simulink model "truck"  (R2022a)
(part 5 of 17)

  M5_erp33360_kros_i_takviyeler_IGS_4_RIGID/LConn1 -- Transform164/RConn1
  M5_erpAynalama3360_kulak_i_takviye_IGS_2_RIGID/LConn1 -- Transform165/RConn1
  M5_erpAynalamaAynalama33360_Kulak_i_L_takviye_IGS_1_RIGID/LConn1 -- Transform166/RConn1
  M5_erp33360_takviye_1_IGS_2_RIGID/LConn1 -- Transform167/RConn1
  M5_erpAynalama33360_kros_ke_takviye_IGS_1_RIGID/LConn1 -- Transform168/RConn1
  M5_erpAynalama33360_kanca_IGS_9_RIGID/LConn1 -- Transform169/RConn1
  Transform17/RConn1 -- mandud_ase_arka_i_destek_1_IGS_1_RIGID/LConn1
  M5_erp33360_takviye_3_IGS_1_RIGID/LConn1 -- Transform170/RConn1
  M5_erp33360_takviye_2_IGS_2_RIGID/LConn1 -- Transform171/RConn1
  M5_erpAynalama33360_kanca_IGS_8_RIGID/LConn1 -- Transform172/RConn1
  M5_erp33360_takviye_2_IGS_1_RIGID/LConn1 -- Transform173/RConn1
  M5_erp33360_takviye_1_IGS_3_RIGID/LConn1 -- Transform174/RConn1
  M5_erpAynalama33360_takviye_3_IGS_1_RIGID/LConn1 -- Transform175/RConn1
  M5_erp3360_kulak_i_takviye_IGS_1_RIGID/LConn1 -- Transform176/RConn1
  M5_erpAynalama33360_takviye_1_IGS_2_RIGID/LConn1 -- Transform177/RConn1
  M5_erp33360_takviye_1_IGS_1_RIGID/LConn1 -- Transform178/RConn1
  M5_erpAynalama33360_takviye_1_IGS_1_RIGID/LConn1 -- Transform179/RConn1
  Transform18/RConn1 -- mandUD_yan_lamba_kablo_borusu_IGS_4_RIGID/LConn1
  M5_erpAynalama33360_takviye_2_IGS_1_RIGID/LConn1 -- Transform180/RConn1
  M5_erpAynalama33360_takviye_2_IGS_2_RIGID/LConn1 -- Transform181/RConn1
  M5_erp33360_kros_ke_takviye_IGS_1_RIGID/LConn1 -- Transform182/RConn1
  M5_erp33360_kros_ke_takviye_IGS_3_RIGID/LConn1 -- Transform183/RConn1
  M5_erp33360_kros_i_takviyeler_IGS_1_RIGID/LConn1 -- Transform184/RConn1
  M5_erp33360_kros_i_takviyeler_IGS_2_RIGID/LConn1 -- Transform185/RConn1
  M5_erp33360_kros_i_takviyeler_IGS_3_RIGID/LConn1 -- Transform186/RConn1
  M5_erp33360_kros_ke_takviye_IGS_4_RIGID/LConn1 -- Transform187/RConn1
  M5_erp33360_merdiven_kula_IGS_2_RIGID/LConn1 -- Transform188/RConn1
  M5_erp33360_merdiven_kula_IGS_5_RIGID/LConn1 -- Transform189/RConn1
  Transform19/RConn1 -- mandud_ase_arka_i_destek_2_IGS_1_RIGID/LConn1
  M5_erpAynalama33360_kros_i_takviyeler_IGS_3_RIGID/LConn1 -- Transform190/RConn1
  M5_erp33360_basamak_IGS_4_RIGID/LConn1 -- Transform191/RConn1
  M5_erp33360_mapa_IGS_2_RIGID/LConn1 -- Transform192/RConn1
  M5_erpAynalama33360_mapa_IGS_2_RIGID/LConn1 -- Transform193/RConn1
  AynalamaM5_erp33360_ZBEKSTAN_ngs_kuak_krosu_IGS_1_RIGID/LConn1 -- Transform194/RConn1
  M5_erp33360_merdiven_kula_IGS_1_RIGID/LConn1 -- Transform195/RConn1
  M5_erp33360_Emniyet_kolu_kasa_paras2_IGS_2_RIGID/LConn1 -- Transform196/RConn1
  M5_erp33360_basamak_IGS_3_RIGID/LConn1 -- Transform197/RConn1
  M5_erp33360_merdiven_kula_IGS_4_RIGID/LConn1 -- Transform198/RConn1
  M5_erpAynalama33360_kros_i_takviyeler_IGS_4_RIGID/LConn1 -- Transform199/RConn1
  Transform2/RConn1 -- x33360_33360_esnek_V_st_para_IGS_1_RIGID/LConn1
  Transform20/RConn1 -- manasi_flan_k8_4_IGS_1_RIGID/LConn1
  M5_erp33360_basamak_IGS_2_RIGID/LConn1 -- Transform200/RConn1
  M5_erp33360_basamak_IGS_5_RIGID/LConn1 -- Transform201/RConn1
  M5_erp33360_merdiven_kenar_IGS_1_RIGID/LConn1 -- Transform202/RConn1
  M5_erp33360_basamak_IGS_6_RIGID/LConn1 -- Transform203/RConn1
  M5_erp33360_basamak_IGS_1_RIGID/LConn1 -- Transform204/RConn1
  M5_erp33360_Emniyet_kolu_kasa_paras1_IGS_1_RIGID/LConn1 -- Transform205/RConn1
  M5_erpAynalama33360_kros_ke_takviye_IGS_2_RIGID/LConn1 -- Transform206/RConn1
  M5_erpAynalama33360_kros_i_takviyeler_IGS_1_RIGID/LConn1 -- Transform207/RConn1
  M5_erpAynalama33360_kros_i_takviyeler_IGS_2_RIGID/LConn1 -- Transform208/RConn1
  M5_erp33360_merdiven_kenar_IGS_2_RIGID/LConn1 -- Transform209/RConn1
  Transform21/RConn1 -- manasi_flan_k8_4_IGS_3_RIGID/LConn1
  M5_erp33360_basamak_IGS_7_RIGID/LConn1 -- Transform210/RConn1
  M5_erp33360_basamak_IGS_8_RIGID/LConn1 -- Transform211/RConn1
  M5_erp33360_merdiven_kula_IGS_3_RIGID/LConn1 -- Transform212/RConn1
  M5_erp33360_Emniyet_kolu_kasa_paras2_IGS_1_RIGID/LConn1 -- Transform213/RConn1
  M5_erp33360_merdiven_kula_IGS_6_RIGID/LConn1 -- Transform214/RConn1
  M5_erp33360_mapa_IGS_1_RIGID/LConn1 -- Transform215/RConn1
  M5_erpAynalama33360_mapa_IGS_1_RIGID/LConn1 -- Transform216/RConn1
  AynalamaM5_erp33360_ZBEKSTAN_kk_yan_kros_IGS_1_RIGID/LConn1 -- Transform217/RConn1
  Kopya_MA_Part_PISTON_GHS_175_5_5550_CM5_Model_004_merkez_IGS_1_/LConn1 -- Transform218/RConn1
  M5_erp33360_n_arka_amurluk_Yeni_Tip_k3_IGS_1_RIGID/LConn1 -- Transform219/RConn1
  Transform22/RConn1 -- manasi_flan_k8_4_IGS_4_RIGID/LConn1
  M5_erp33360_siperlik_IGS_1_RIGID/LConn1 -- Transform220/RConn1
  M5_erp33360_KMS_298_IGS_1_RIGID/LConn1 -- Transform221/RConn1
  M5_erp33360_Aynalamaamurluk_aya_kebenti_6mm_IGS_3_RIGID/LConn1 -- Transform222/RConn1
  M5_erp33360_amurluk_aya_kebenti_6mm_IGS_1_RIGID/LConn1 -- Transform223/RConn1
  M5_erp33360_KMS_207_IGS_1_RIGID/LConn1 -- Transform224/RConn1
  M5_erp33360_Aynalamaamurluk_aya_kebenti_6mm_IGS_4_RIGID/LConn1 -- Transform225/RConn1
  M5_erp33360_KMS_298_IGS_2_RIGID/LConn1 -- Transform226/RConn1
  M5_erp33360_Aynalamai_kaytr_IGS_1_RIGID/LConn1 -- Transform227/RConn1
  M5_erp33360_KMK_226_IGS_1_RIGID/LConn1 -- Transform228/RConn1
  M5_erp33360_ase_kamaz_6_mm_IGS_1_RIGID/LConn1 -- Transform229/RConn1
  Transform23/RConn1 -- manasi_flan_k8_4_IGS_2_RIGID/LConn1
  M5_erp33360_KMS_202_IGS_2_RIGID/LConn1 -- Transform230/RConn1
  M5_erp33360_KMS_202_IGS_3_RIGID/LConn1 -- Transform231/RConn1
  M5_erp33360_siperlik_yan_sac_IGS_1_RIGID/LConn1 -- Transform232/RConn1
  M5_erp33360_KMS_202_IGS_1_RIGID/LConn1 -- Transform233/RConn1
  M5_erp33360_Aynalamaamurluk_aya_kebenti_6mm_IGS_2_RIGID/LConn1 -- Transform234/RConn1
  M5_erp33360_ase_kamaz_6_mm_IGS_2_RIGID/LConn1 -- Transform235/RConn1
  M5_erp33360_Aynalamasiperlik_yan_sac_IGS_1_RIGID/LConn1 -- Transform236/RConn1
  M5_erp33360_KMS_202_IGS_4_RIGID/LConn1 -- Transform237/RConn1
  M5_erp33360_kros_kebent_IGS_1_RIGID/LConn1 -- Transform238/RConn1
  M5_erp33360_amurluk_aya_kk_kebent_6mm_IGS_1_RIGID/LConn1 -- Transform239/RConn1
  Transform24/RConn1 -- manpistonaltbaskstsac_k10_1_IGS_1_RIGID/LConn1
  M5_erp33360_Aynalamaamurluk_aya_kebenti_6mm_IGS_1_RIGID/LConn1 -- Transform240/RConn1
  M5_erp33360_HD_654_IGS_1_RIGID/LConn1 -- Transform241/RConn1
  M5_erp33360_ase_kamaz_arka_sac_6mm_IGS_1_RIGID/LConn1 -- Transform242/RConn1
  M5_erpAynalama33360_KMS_202_IGS_2_RIGID/LConn1 -- Transform243/RConn1
  M5_erpAynalama33360_KMS_202_IGS_4_RIGID/LConn1 -- Transform244/RConn1
  M5_erpAynalama33360_KMK_236_IGS_1_RIGID/LConn1 -- Transform245/RConn1
  M5_erp33360_siperlik_lamas_IGS_1_RIGID/LConn1 -- Transform246/RConn1
  M5_erpAynalama33360_KMS_207_IGS_1_RIGID/LConn1 -- Transform247/RConn1
  M5_erpAynalama33360_Aynalamaamurluk_aya_kebenti_6mm_IGS_1_RIGID/LConn1 -- Transform248/RConn1
  M5_erpAynalama33360_amurluk_sac_k4_IGS_1_RIGID/LConn1 -- Transform249/RConn1
  Transform25/RConn1 -- mandAynalamaUD_altbask_i_IGS_1_RIGID/LConn1
  M5_erp33360_Aynalamanpanel_dke_takviyesi_IGS_1_RIGID/LConn1 -- Transform250/RConn1
  M5_erpAynalama33360_KMS_202_IGS_3_RIGID/LConn1 -- Transform251/RConn1
  M5_erpAynalama33360_KMS_202_IGS_1_RIGID/LConn1 -- Transform252/RConn1
  M5_erp33360_npanel_dke_takviyesi_IGS_1_RIGID/LConn1 -- Transform253/RConn1
  M5_erpAynalama33360_i_amurluk_aya_k6_IGS_2_RIGID/LConn1 -- Transform254/RConn1
  M5_erpAynalama33360_i_amurluk_aya_paspas_gelenler_IGS_1_RIGID/LConn1 -- Transform255/RConn1
  M5_erpAynalama33360_n_arka_amurluk_Yeni_Tip_k3_IGS_1_RIGID/LConn1 -- Transform256/RConn1
  M5_erp33360_i_sehim_takviyesi_IGS_1_RIGID/LConn1 -- Transform257/RConn1
  M5_erpAynalama33360_i_amurluk_aya_k6_IGS_1_RIGID/LConn1 -- Transform258/RConn1
  M5_erp33360_npanel_ike_takviyesi_IGS_1_RIGID/LConn1 -- Transform259/RConn1
  Transform26/RConn1 -- mandUD_altbask_i_IGS_1_RIGID/LConn1
  M5_erpAynalama33360_n_amurluk_aya_k6_IGS_1_RIGID/LConn1 -- Transform260/RConn1
  M5_erpAynalama33360_npanel_ike_takviyesi_IGS_1_RIGID/LConn1 -- Transform261/RConn1
  M5_erp33360_n_arka_amurluk_Yeni_Tip_k3_IGS_2_RIGID/LConn1 -- Transform262/RConn1
  M5_erp33360_i_sehim_takviyesi_IGS_2_RIGID/LConn1 -- Transform263/RConn1
  M5_erpAynalama33360_arka_amurluk_aya_6mm_IGS_1_RIGID/LConn1 -- Transform264/RConn1
  M5_erpAynalama33360_i_amurluk_aya_paspas_gelenler_IGS_2_RIGID/LConn1 -- Transform265/RConn1
  M5_erpAynalama33360_n_arka_amurluk_Yeni_Tip_k3_IGS_2_RIGID/LConn1 -- Transform266/RConn1
  M5_erpAynalama33360_HD_654_IGS_1_RIGID/LConn1 -- Transform267/RConn1
  M5_erpAynalama33360_KMK_226_IGS_1_RIGID/LConn1 -- Transform268/RConn1
  M5_erpAynalama33360_KMS_298_IGS_1_RIGID/LConn1 -- Transform269/RConn1
  Transform27/RConn1 -- mandUD_ya_tank_aya_destek_IGS_1_RIGID/LConn1
  M5_erpAynalama33360_KMS_298_IGS_2_RIGID/LConn1 -- Transform270/RConn1
  M5_erpAynalama33360_kros_kebent_IGS_1_RIGID/LConn1 -- Transform271/RConn1
  M5_erpAynalama33360_Aynalamaamurluk_aya_kebenti_6mm_IGS_2_RIGID/LConn1 -- Transform272/RConn1
  M5_erpAynalama33360_amurluk_aya_kk_kebent_6mm_IGS_1_RIGID/LConn1 -- Transform273/RConn1
  M5_erpAynalama33360_ase_kamaz_6_mm_IGS_1_RIGID/LConn1 -- Transform274/RConn1
  M5_erpAynalama33360_ase_kamaz_arka_sac_6mm_IGS_1_RIGID/LConn1 -- Transform275/RConn1
  M5_erpAynalama33360_Aynalamaamurluk_aya_kebenti_6mm_IGS_4_RIGID/LConn1 -- Transform276/RConn1
  M5_erpAynalama33360_amurluk_aya_kebenti_6mm_IGS_1_RIGID/LConn1 -- Transform277/RConn1
  M5_erp33360_ikayt_arka_kaama_IGS_1_RIGID/LConn1 -- Transform278/RConn1
  M5_erpAynalama33360_ikayt_arka_kaama_IGS_1_RIGID/LConn1 -- Transform279/RConn1
  Transform28/RConn1 -- mandUD_yan_lamba_kablo_borusu_IGS_1_RIGID/LConn1
  M5_erpAynalama33360_ase_kamaz_6_mm_IGS_2_RIGID/LConn1 -- Transform280/RConn1
  M5_erp33360_kapak_IGS_1_RIGID/LConn1 -- Transform281/RConn1
  M5_erpAynalama33360_Aynalamaamurluk_aya_kebenti_6mm_IGS_3_RIGID/LConn1 -- Transform282/RConn1
  Transform283/RConn1 -- x33360_pulll_IGS_9_RIGID/LConn1
  Transform284/RConn1 -- x33360_33360_esnek_V_st_para_IGS_2_RIGID/LConn1
  Transform285/RConn1 -- x33360_pulll_IGS_12_RIGID/LConn1
  Transform286/RConn1 -- x33360_23658911_IGS_3_RIGID/LConn1
  Transform287/RConn1 -- x33360_23658911_IGS_5_RIGID/LConn1
  Transform288/RConn1 -- x33360_23658911_IGS_7_RIGID/LConn1
  Transform289/RConn1 -- x33360_esnek_baglanti_poliuretan_takoz_IGS_2_RIGID/LConn1
  Transform29/RConn1 -- ayakflan_k8_4_IGS_2_RIGID/LConn1
  Transform290/RConn1 -- x33360_33360_2li_esnke_ara_para_IGS_2_RIGID/LConn1
  Transform291/RConn1 -- x33360_HEX_NUT_ISO_8673_M16_X_1_5_IGS_3_RIGID/LConn1
  Transform292/RConn1 -- x33360_23658911_IGS_6_RIGID/LConn1
  Transform293/RConn1 -- x33360_33360_2li_esnke_ara_para_IGS_1_RIGID/LConn1
  Transform294/RConn1 -- x33360_pulll_IGS_2_RIGID/LConn1
  Transform295/RConn1 -- x33360_pulll_IGS_4_RIGID/LConn1
  Transform296/RConn1 -- x33360_pulll_IGS_8_RIGID/LConn1
  Transform297/RConn1 -- x33360_33360_esnek_ust_ped_IGS_1_RIGID/LConn1
  Transform298/RConn1 -- x33360_pulll_IGS_6_RIGID/LConn1
  Transform299/RConn1 -- x33360_33360_Esnek_V_alt_para_uzun_IGS_1_RIGID/LConn1
  M33360_26280_mil_no8_IGS_1_RIGID/LConn1 -- Transform3/RConn1
  Transform30/RConn1 -- ayakflan_k8_4_IGS_3_RIGID/LConn1
  Transform300/RConn1 -- x33360_pulll_IGS_3_RIGID/LConn1
  Transform301/RConn1 -- x33360_33360_esnek_ust_ped_IGS_2_RIGID/LConn1
  Transform302/RConn1 -- x33360_pulll_IGS_5_RIGID/LConn1
  Transform303/RConn1 -- x33360_pulll_IGS_7_RIGID/LConn1
  Transform304/RConn1 -- x33360_33360_ESNEK_UZUN_ALT_PED_IGS_1_RIGID/LConn1
  Transform305/RConn1 -- x33360_pulll_IGS_10_RIGID/LConn1
  Transform306/RConn1 -- x33360_pulll_IGS_1_RIGID/LConn1
  Transform307/RConn1 -- x33360_pulll_IGS_11_RIGID/LConn1
  Transform308/RConn1 -- x33360_23658911_IGS_1_RIGID/LConn1
  Transform309/RConn1 -- x33360_23658911_IGS_2_RIGID/LConn1
  Transform31/RConn1 -- x132zbmut4900zT13124_ozaas_Part2_IGS_1_RIGID/LConn1
  Transform310/RConn1 -- x33360_23658911_IGS_4_RIGID/LConn1
  Transform311/RConn1 -- x33360_23658911_IGS_8_RIGID/LConn1
  Transform312/RConn1 -- x33360_esnek_baglanti_poliuretan_takoz_IGS_1_RIGID/LConn1
  Transform313/RConn1 -- x33360_HEX_NUT_ISO_8673_M16_X_1_5_IGS_1_RIGID/LConn1
  Transform314/RConn1 -- x33360_HEX_NUT_ISO_8673_M16_X_1_5_IGS_2_RIGID/LConn1
  Aynalama33360_33360_esnek_V_st_para_IGS_2_RIGID/LConn1 -- Transform315/RConn1
  Transform316/RConn1 -- x33360_burlu_balant_burcu_IGS_2_RIGID/LConn1
  Aynalama33360_pulll_IGS_1_RIGID/LConn1 -- Transform317/RConn1
  Transform318/RConn1 -- x33360_HEX_NUT_ISO_8673_M16_X_1_5_IGS_4_RIGID/LConn1
  Aynalama33360_33360_2li_esnke_ara_para_IGS_2_RIGID/LConn1 -- Transform319/RConn1
  Transform32/RConn1 -- x132zbmut4900zT13124_ozaas_Part2_IGS_2_RIGID/LConn1
  Aynalama33360_pulll_IGS_8_RIGID/LConn1 -- Transform320/RConn1
  Aynalama33360_pulll_IGS_5_RIGID/LConn1 -- Transform321/RConn1
  Transform322/RConn1 -- x33360_KMS_305_IGS_1_RIGID/LConn1
  Son_model_3_IGS_3_RIGID/LConn1 -- Transform323/RConn1
  Aynalama33360_esnek_baglanti_poliuretan_takoz_IGS_1_RIGID/LConn1 -- Transform324/RConn1
  Transform325/RConn1 -- x33360_MS_009_IGS_1_RIGID/LConn1
  Aynalama33360_pulll_IGS_2_RIGID/LConn1 -- Transform326/RConn1
  Aynalama33360_esnek_baglanti_poliuretan_takoz_IGS_2_RIGID/LConn1 -- Transform327/RConn1
  Aynalama33360_pulll_IGS_11_RIGID/LConn1 -- Transform328/RConn1
  Transform329/RConn1 -- x33360_burlu_balant_burcu_IGS_1_RIGID/LConn1
  Ayak_Sac3_752_IGS_1_RIGID/LConn1 -- Transform33/RConn1
  Aynalama33360_33360_Esnek_V_alt_para_uzun_IGS_1_RIGID/LConn1 -- Transform330/RConn1
  Aynalama33360_33360_2li_esnke_ara_para_IGS_1_RIGID/LConn1 -- Transform331/RConn1
  Aynalama33360_33360_esnek_ust_ped_IGS_2_RIGID/LConn1 -- Transform332/RConn1
  Transform333/RConn1 -- x33360_arkamilbalant_IGS_1_RIGID/LConn1
  Son_model_3_IGS_1_RIGID/LConn1 -- Transform334/RConn1
  Aynalama33360_33360_ESNEK_UZUN_ALT_PED_IGS_1_RIGID/LConn1 -- Transform335/RConn1
  Transform336/RConn1 -- x33360_MS_008_IGS_1_RIGID/LConn1
  Son_model_3_IGS_2_RIGID/LConn1 -- Transform337/RConn1
  Aynalama33360_33360_esnek_V_st_para_IGS_1_RIGID/LConn1 -- Transform338/RConn1
  Aynalama33360_33360_esnek_ust_ped_IGS_1_RIGID/LConn1 -- Transform339/RConn1
  Transform34/RConn1 -- ayakflan_k8_4_IGS_1_RIGID/LConn1
  Aynalama33360_pulll_IGS_3_RIGID/LConn1 -- Transform340/RConn1
  Aynalama33360_pulll_IGS_4_RIGID/LConn1 -- Transform341/RConn1
  Aynalama33360_pulll_IGS_6_RIGID/LConn1 -- Transform342/RConn1
  Aynalama33360_pulll_IGS_7_RIGID/LConn1 -- Transform343/RConn1
  Aynalama33360_pulll_IGS_9_RIGID/LConn1 -- Transform344/RConn1
  Aynalama33360_pulll_IGS_10_RIGID/LConn1 -- Transform345/RConn1
  Aynalama33360_pulll_IGS_12_RIGID/LConn1 -- Transform346/RConn1
  Aynalama33360_HEX_NUT_ISO_8673_M16_X_1_5_IGS_4_RIGID/LConn1 -- Transform347/RConn1
  Transform348/RConn1 -- st_kapama_L_ayak_sasi_paras_21_IGS_2_RIGID/LConn1
  AynalamaSon_model_3_IGS_1_RIGID/LConn1 -- Transform349/RConn1
  Ayak_Sac4_692_IGS_1_RIGID/LConn1 -- Transform35/RConn1
  Transform350/RConn1 -- ayakl_flans_IGS_1_RIGID/LConn1
  Ayak_U_ase_paras_IGS_1_RIGID/LConn1 -- Transform351/RConn1
  Transform352/RConn1 -- st_kapama_L_ayak_sasi_paras_21_IGS_1_RIGID/LConn1
  Transform353/RConn1 -- YAPI_plastik_cmurluk_bru_ust_bayrak_IGS_2_RIGID/LConn1
  Aynalama33360_MS_008_IGS_1_RIGID/LConn1 -- Transform354/RConn1
  AynalamaYAPI_plastik_cmurluk_bru_ust_bayrak_IGS_4_RIGID/LConn1 -- Transform355/RConn1
  AynalamaYAPI_plastik_camurluk_IGS_2_RIGID/LConn1 -- Transform356/RConn1
  Aynalamaayakl_flans_IGS_1_RIGID/LConn1 -- Transform357/RConn1
  Aynalamast_kapama_L_ayak_sasi_paras_21_IGS_1_RIGID/LConn1 -- Transform358/RConn1
  Aynalama33360_MS_009_IGS_1_RIGID/LConn1 -- Transform359/RConn1
  Transform36/RConn1 -- x132zbmut4900zT13124_ozaas_Part2_IGS_3_RIGID/LConn1
  Aynalama33360_burlu_balant_burcu_IGS_1_RIGID/LConn1 -- Transform360/RConn1
  Aynalama33360_arkamilbalant_IGS_1_RIGID/LConn1 -- Transform361/RConn1
  Plastik_amurluk_st_kapama1_IGS_1_RIGID/LConn1 -- Transform362/RConn1
  AynalamaYAPI_plastik_cmurluk_bru_ust_bayrak_IGS_1_RIGID/LConn1 -- Transform363/RConn1
  Aynalama33360_HEX_NUT_ISO_8673_M16_X_1_5_IGS_1_RIGID/LConn1 -- Transform364/RConn1
  Aynalama33360_HEX_NUT_ISO_8673_M16_X_1_5_IGS_3_RIGID/LConn1 -- Transform365/RConn1
  Aynalama33360_burlu_balant_burcu_IGS_2_RIGID/LConn1 -- Transform366/RConn1
  AynalamaSon_model_3_IGS_3_RIGID/LConn1 -- Transform367/RConn1
  AynalamaSon_model_3_IGS_2_RIGID/LConn1 -- Transform368/RConn1
  Ayak_U_ase_paras_IGS_2_RIGID/LConn1 -- Transform369/RConn1
  Transform37/RConn1 -- x132zbmut4900zT13124_ozaas_Part2_IGS_4_RIGID/LConn1
  Aynalama33360_HEX_NUT_ISO_8673_M16_X_1_5_IGS_2_RIGID/LConn1 -- Transform370/RConn1
  Transform371/RConn1 -- ayakl_flans_IGS_2_RIGID/LConn1
  Transform372/RConn1 -- YAPI_plastik_cmurluk_bru_ust_bayrak_IGS_1_RIGID/LConn1
  Transform373/RConn1 -- YAPI_boruu_IGS_1_RIGID/LConn1
  Transform374/RConn1 -- YAPI_plastik_camurluk_IGS_1_RIGID/LConn1
  AynalamaYAPI_boruu_IGS_1_RIGID/LConn1 -- Transform375/RConn1
  AynalamaYAPI_boruu_IGS_2_RIGID/LConn1 -- Transform376/RConn1
  AynalamaYAPI_plastik_cmurluk_bru_ust_bayrak_IGS_2_RIGID/LConn1 -- Transform377/RConn1
  AynalamaYAPI_plastik_cmurluk_bru_ust_bayrak_IGS_3_RIGID/LConn1 -- Transform378/RConn1
  AynalamaYAPI_plastik_camurluk_IGS_1_RIGID/LConn1 -- Transform379/RConn1
  Transform38/RConn1 -- x132zbmut4900zT13124_ozaas_Part1_IGS_1_RIGID/LConn1
  AynalamaPlastik_amurluk_st_kapama1_IGS_1_RIGID/LConn1 -- Transform380/RConn1
  Aynalamaayakl_flans_IGS_2_RIGID/LConn1 -- Transform381/RConn1
  M5_erp33360_KMK_214_IGS_1_RIGID/LConn1 -- Transform382/RConn1
  M5_erp33360_HD_604_IGS_2_RIGID/LConn1 -- Transform383/RConn1
  M5_erp33360_HDS_607_IGS_1_RIGID/LConn1 -- Transform384/RConn1
  M5_erp33360_ZBEKSTAN_kulak_krosu_IGS_1_RIGID/LConn1 -- Transform385/RConn1
  M5_erp33360_ZBEKSTAN_n_dikme_IGS_1_RIGID/LConn1 -- Transform386/RConn1
  M5_erp33360_KMK_213_IGS_1_RIGID/LConn1 -- Transform387/RConn1
  M5_erp33360_YAN_6_MM_ST_IGS_1_RIGID/LConn1 -- Transform388/RConn1
  M5_erp33360_ZBEKSTAN_Byk_Yan_Kros_IGS_1_RIGID/LConn1 -- Transform389/RConn1
  Ayak_Sac1_627_IGS_1_RIGID/LConn1 -- Transform39/RConn1
  AynalamaAyak_U_ase_paras_IGS_1_RIGID/LConn1 -- Transform390/RConn1
  M5_erp33360_HD_601_IGS_1_RIGID/LConn1 -- Transform391/RConn1
  M5_erp33360_ZBEKSTAN_kk_yan_kros_IGS_1_RIGID/LConn1 -- Transform392/RConn1
  M5_erp33360_HD_604_IGS_1_RIGID/LConn1 -- Transform393/RConn1
  M5_erp33360_HDS_606_IGS_1_RIGID/LConn1 -- Transform394/RConn1
  AynalamaAynalamaYAPI_plastik_cmurluk_bru_ust_bayrak_IGS_1_RIGID/LConn1 -- Transform395/RConn1
  M5_erp33360_TABAN_8_MM_ST_IGS_1_RIGID/LConn1 -- Transform396/RConn1
  M5_erp33360_HD_602_IGS_1_RIGID/LConn1 -- Transform397/RConn1
  AynalamaAynalamaYAPI_plastik_camurluk_IGS_1_RIGID/LConn1 -- Transform398/RConn1
  M5_erp33360_ZBEKSTAN_En_Arka_Taban_Krosu_IGS_1_RIGID/LConn1 -- Transform399/RConn1
  M33360_26280_para_no6_IGS_1_RIGID/LConn1 -- Transform4/RConn1
  Transform40/RConn1 -- ayakflan_k8_4_IGS_4_RIGID/LConn1
  Aynalamast_kapama_L_ayak_sasi_paras_21_IGS_2_RIGID/LConn1 -- Transform400/RConn1
  M5_erp33360_NPANEL_6_MM_ST_IGS_1_RIGID/LConn1 -- Transform401/RConn1
  AynalamaAyak_U_ase_paras_IGS_2_RIGID/LConn1 -- Transform402/RConn1
  AynalamaAynalamaYAPI_boruu_IGS_1_RIGID/LConn1 -- Transform403/RConn1
  AynalamaAynalamaYAPI_plastik_cmurluk_bru_ust_bayrak_IGS_2_RIGID/LConn1 -- Transform404/RConn1
  M5_erp33360_MirrorYAN_6_MM_ST_IGS_1_RIGID/LConn1 -- Transform405/RConn1
  M5_erp33360_KMK_214_IGS_2_RIGID/LConn1 -- Transform406/RConn1
  M5_erp33360_KMK_213_IGS_2_RIGID/LConn1 -- Transform407/RConn1
  M5_erp33360_HDS_608_IGS_1_RIGID/LConn1 -- Transform408/RConn1
  M5_erp33360_ZBEKSTAN_ngs_kuak_krosu_IGS_1_RIGID/LConn1 -- Transform409/RConn1
  Ayak_Sac2_642_IGS_1_RIGID/LConn1 -- Transform41/RConn1
  M5_erp33360_i_kaytr_IGS_1_RIGID/LConn1 -- Transform410/RConn1
  M5_erp33360_ZBEKSTAN_kilit_takviye_2_IGS_1_RIGID/LConn1 -- Transform411/RConn1
  M5_erp33360_AynalamaZBEKSTAN_kilit_krosu_bayrak_IGS_1_RIGID/LConn1 -- Transform412/RConn1
  M5_erp33360_amurluk_sac_k4_IGS_1_RIGID/LConn1 -- Transform413/RConn1
  M5_erp33360_MirrorZBEKSTAN_Byk_Yan_Kros_IGS_1_RIGID/LConn1 -- Transform414/RConn1
  M5_erp33360_MirrorZBEKSTAN_n_dikme_IGS_1_RIGID/LConn1 -- Transform415/RConn1
  M5_erp33360_n_amurluk_aya_k6_IGS_1_RIGID/LConn1 -- Transform416/RConn1
  M5_erp33360_i_amurluk_aya_k6_IGS_1_RIGID/LConn1 -- Transform417/RConn1
  M5_erp33360_i_amurluk_aya_k6_IGS_2_RIGID/LConn1 -- Transform418/RConn1
  M5_erp33360_ZBEKSTAN_kilit_krosu_bayrak_IGS_1_RIGID/LConn1 -- Transform419/RConn1
  Transform42/RConn1 -- x132zbmut4900zT13124_ozaas_Part1_IGS_2_RIGID/LConn1
  M5_erp33360_arka_amurluk_aya_6mm_IGS_1_RIGID/LConn1 -- Transform420/RConn1
  M5_erp33360_i_amurluk_aya_paspas_gelenler_IGS_1_RIGID/LConn1 -- Transform421/RConn1
  M5_erp33360_i_amurluk_aya_paspas_gelenler_IGS_2_RIGID/LConn1 -- Transform422/RConn1
  M5_erp33360_KMK_236_IGS_1_RIGID/LConn1 -- Transform423/RConn1
  M5_Model_004_merkez_10_1_IGS_1_RIGID/LConn1 -- Transform424/RConn1
  M5_Model_004_Basit_Travers_IGS_1_RIGID/LConn1 -- Transform425/RConn1
  M5_Model_004_merkez_2_IGS_1_RIGID/LConn1 -- Transform426/RConn1
  M5_Model_004_merkez_3_1_IGS_1_RIGID/LConn1 -- Transform427/RConn1
  M5_Model_004_merkez_2_1_IGS_1_RIGID/LConn1 -- Transform428/RConn1
  M5_Model_004_merkez_4_1_IGS_1_RIGID/LConn1 -- Transform429/RConn1
  M5_Model_004_Ayna_01_IGS_1_RIGID/LConn1 -- Transform43/RConn1
  M5_Model_004_merkez_1_1_IGS_1_RIGID/LConn1 -- Transform430/RConn1
  M5_Model_004_merkez_5_1_IGS_1_RIGID/LConn1 -- Transform431/RConn1
  M5_Model_004_merkez_6_1_IGS_1_RIGID/LConn1 -- Transform432/RConn1
  M5_Model_004_merkez_7_1_IGS_1_RIGID/LConn1 -- Transform433/RConn1
  M5_Model_004_merkez_8_1_IGS_1_RIGID/LConn1 -- Transform434/RConn1
  M5_Model_004_merkez_9_1_IGS_1_RIGID/LConn1 -- Transform435/RConn1
  M5_Model_004_merkez_11_1_IGS_1_RIGID/LConn1 -- Transform436/RConn1
  M5_Model_004_Basit_Travers_IGS_3_RIGID/LConn1 -- Transform437/RConn1
  M5_Jant_IGS_9_RIGID/LConn1 -- Transform438/RConn1
  M5_Lastik_IGS_2_RIGID/LConn1 -- Transform439/RConn1
  M5_Model_004_05_1_IGS_1_RIGID/LConn1 -- Transform44/RConn1
  M5_Model_004_1_03_IGS_1_RIGID/LConn1 -- Transform440/RConn1
  M5_Jant_IGS_8_RIGID/LConn1 -- Transform441/RConn1
  M5_Model_004_1_03_IGS_2_RIGID/LConn1 -- Transform442/RConn1
  M5_Lastik_IGS_8_RIGID/LConn1 -- Transform443/RConn1
  Part1M5_Model_004_merkez_IGS_1_RIGID/LConn1 -- Transform444/RConn1
  M5_Model_004_Basit_Travers_IGS_2_RIGID/LConn1 -- Transform445/RConn1
  M5_Jant_IGS_4_RIGID/LConn1 -- Transform446/RConn1
  M5_Lastik_IGS_7_RIGID/LConn1 -- Transform447/RConn1
  M5_Model_003_kapak_ks_versiyon_IGS_1_RIGID/LConn1 -- Transform448/RConn1
  M5_Model_003_kapak_ks_versiyon_IGS_3_RIGID/LConn1 -- Transform449/RConn1
  M5_MirrorUV_01_IGS_1_RIGID/LConn1 -- Transform45/RConn1
  M5_Jant_IGS_6_RIGID/LConn1 -- Transform450/RConn1
  M5_Jant_IGS_2_RIGID/LConn1 -- Transform451/RConn1
  M5_Lastik_IGS_1_RIGID/LConn1 -- Transform452/RConn1
  M5_Lastik_IGS_9_RIGID/LConn1 -- Transform453/RConn1
  M5_Jant_IGS_1_RIGID/LConn1 -- Transform454/RConn1
  M5_Jant_IGS_5_RIGID/LConn1 -- Transform455/RConn1
  M5_Jant_IGS_10_RIGID/LConn1 -- Transform456/RConn1
  M5_Jant_IGS_7_RIGID/LConn1 -- Transform457/RConn1
  M5_Lastik_IGS_4_RIGID/LConn1 -- Transform458/RConn1
  M5_Lastik_IGS_3_RIGID/LConn1 -- Transform459/RConn1
  Transform46/RConn1 -- mandUD_Hekimhan_Madencilik_ergnler_3028U_ase_IGS_1_RIGID/LConn1
  M5_Jant_IGS_3_RIGID/LConn1 -- Transform460/RConn1
  M5_Lastik_IGS_5_RIGID/LConn1 -- Transform461/RConn1
  M5_Lastik_IGS_6_RIGID/LConn1 -- Transform462/RConn1
  M5_Lastik_IGS_10_RIGID/LConn1 -- Transform463/RConn1
  M5_Model_004_1_03_IGS_3_RIGID/LConn1 -- Transform464/RConn1
  M5_Model_004_1_03_IGS_4_RIGID/LConn1 -- Transform465/RConn1
  M5_Model_004_1_03_IGS_5_RIGID/LConn1 -- Transform466/RConn1
  M5_Model_004_1_03_IGS_6_RIGID/LConn1 -- Transform467/RConn1
  Part1M5_Model_004_merkez_IGS_2_RIGID/LConn1 -- Transform468/RConn1
  Part1M5_Model_004_merkez_IGS_3_RIGID/LConn1 -- Transform469/RConn1
  Part4M5_Model_004_merkez_IGS_1_RIGID/LConn1 -- Transform47/RConn1
  M5_Model_003_kapak_IGS_1_RIGID/LConn1 -- Transform470/RConn1
  M5_Model_003_kapak_IGS_2_RIGID/LConn1 -- Transform471/RConn1
  M5_Model_003_kapak_ks_versiyon_IGS_2_RIGID/LConn1 -- Transform472/RConn1
  M5_Model_003_kapak_ks_versiyon_IGS_4_RIGID/LConn1 -- Transform473/RConn1
  Transform/LConn1 -- Transform98/LConn1 -- Transform99/LConn1 -- Transform97/LConn1 -- Transform96/LConn1 -- Transform95/LConn1 -- Transform94/LConn1 -- Transform93/LConn1 -- Transform92/LConn1 -- Transform91/LConn1 -- Transform90/LConn1 -- Transform9/LConn1 -- Transform89/LConn1 -- Transform88/LConn1 -- Transform87/LConn1 -- Transform86/LConn1 -- Transform85/LConn1 -- Transform84/LConn1 -- Transform83/LConn1 -- Transform82/LConn1 -- Transform81/LConn1 -- Transform80/LConn1 -- Transform8/LConn1 -- Transform79/LConn1 -- Transform78/LConn1 -- Transform77/LConn1 -- Transform76/LConn1 -- Transform75/LConn1 -- Transform74/LConn1 -- Transform73/LConn1 -- Transform72/LConn1 -- Transform71/LConn1 -- Transform70/LConn1 -- Transform7/LConn1 -- Transform69/LConn1 -- Transform68/LConn1 -- Transform67/LConn1 -- Transform66/LConn1 -- Transform65/LConn1 -- Transform64/LConn1 -- Transform63/LConn1 -- Transform62/LConn1 -- Transform61/LConn1 -- Transform60/LConn1 -- Transform6/LConn1 -- Transform59/LConn1 -- Transform58/LConn1 -- Transform57/LConn1 -- Transform56/LConn1 -- Transform55/LConn1 -- Transform54/LConn1 -- Transform53/LConn1 -- Transform52/LConn1 -- Transform51/LConn1 -- Transform50/LConn1 -- Transform5/LConn1 -- Transform49/LConn1 -- Transform48/LConn1 -- Transform473/LConn1 -- Transform472/LConn1 -- Transform471/LConn1 -- Transform470/LConn1 -- Transform47/LConn1 -- Transform469/LConn1 -- Transform468/LConn1 -- Transform467/LConn1 -- Transform466/LConn1 -- Transform465/LConn1 -- Transform464/LConn1 -- Transform463/LConn1 -- Transform462/LConn1 -- Transform461/LConn1 -- Transform460/LConn1 -- Transform46/LConn1 -- Transform459/LConn1 -- Transform458/LConn1 -- Transform457/LConn1 -- Transform456/LConn1 -- Transform455/LConn1 -- Transform454/LConn1 -- Transform453/LConn1 -- Transform452/LConn1 -- Transform451/LConn1 -- Transform450/LConn1 -- Transform45/LConn1 -- Transform449/LConn1 -- Transform448/LConn1 -- Transform447/LConn1 -- Transform446/LConn1 -- Transform445/LConn1 -- Transform444/LConn1 -- Transform443/LConn1 -- Transform442/LConn1 -- Transform441/LConn1 -- Transform440/LConn1 -- Transform44/LConn1 -- Transform439/LConn1 -- Transform438/LConn1 -- Transform437/LConn1 -- Transform436/LConn1 -- Transform435/LConn1 -- Transform434/LConn1 -- Transform433/LConn1 -- Transform432/LConn1 -- Transform431/LConn1 -- Transform430/LConn1 -- Transform43/LConn1 -- Transform429/LConn1 -- Transform428/LConn1 -- Transform427/LConn1 -- Transform426/LConn1 -- Transform425/LConn1 -- Transform424/LConn1 -- Transform423/LConn1 -- Transform422/LConn1 -- Transform421/LConn1 -- Transform420/LConn1 -- Transform42/LConn1 -- Transform419/LConn1 -- Transform418/LConn1 -- Transform417/LConn1 -- Transform416/LConn1 -- Transform415/LConn1 -- Transform414/LConn1 -- Transform413/LConn1 -- Transform412/LConn1 -- Transform411/LConn1 -- Transform410/LConn1 -- Transform41/LConn1 -- Transform409/LConn1 -- Transform408/LConn1 -- Transform407/LConn1 -- Transform406/LConn1 -- Transform405/LConn1 -- Transform404/LConn1 -- Transform403/LConn1 -- Transform402/LConn1 -- Transform401/LConn1 -- Transform400/LConn1 -- Transform40/LConn1 -- Transform4/LConn1 -- Transform399/LConn1 -- Transform398/LConn1 -- Transform397/LConn1 -- Transform396/LConn1 -- Transform395/LConn1 -- Transform394/LConn1 -- Transform393/LConn1 -- Transform392/LConn1 -- Transform391/LConn1 -- Transform390/LConn1 -- Transform39/LConn1 -- Transform389/LConn1 -- Transform388/LConn1 -- Transform387/LConn1 -- Transform386/LConn1 -- Transform385/LConn1 -- Transform384/LConn1 -- Transform383/LConn1 -- Transform382/LConn1 -- Transform381/LConn1 -- Transform380/LConn1 -- Transform38/LConn1 -- Transform379/LConn1 -- Transform378/LConn1 -- Transform377/LConn1 -- Transform376/LConn1 -- Transform375/LConn1 -- Transform374/LConn1 -- Transform373/LConn1 -- Transform372/LConn1 -- Transform371/LConn1 -- Transform370/LConn1 -- Transform37/LConn1 -- Transform369/LConn1 -- Transform368/LConn1 -- Transform367/LConn1 -- Transform366/LConn1 -- Transform365/LConn1 -- Transform364/LConn1 -- Transform363/LConn1 -- Transform362/LConn1 -- Transform361/LConn1 -- Transform360/LConn1 -- Transform36/LConn1 -- Transform359/LConn1 -- Transform358/LConn1 -- Transform357/LConn1 -- Transform356/LConn1 -- Transform355/LConn1 -- Transform354/LConn1 -- Transform353/LConn1 -- Transform352/LConn1 -- Transform351/LConn1 -- Transform350/LConn1 -- Transform35/LConn1 -- Transform349/LConn1 -- Transform348/LConn1 -- Transform347/LConn1 -- Transform346/LConn1 -- Transform345/LConn1 -- Transform344/LConn1 -- Transform343/LConn1 -- Transform342/LConn1 -- Transform341/LConn1 -- Transform340/LConn1 -- Transform34/LConn1 -- Transform339/LConn1 -- Transform338/LConn1 -- Transform337/LConn1 -- Transform336/LConn1 -- Transform335/LConn1 -- Transform334/LConn1 -- Transform333/LConn1 -- Transform332/LConn1 -- Transform331/LConn1 -- Transform330/LConn1 -- Transform33/LConn1 -- Transform329/LConn1 -- Transform328/LConn1 -- Transform327/LConn1 -- Transform326/LConn1 -- Transform325/LConn1 -- Transform324/LConn1 -- Transform323/LConn1 -- Transform322/LConn1 -- Transform321/LConn1 -- Transform320/LConn1 -- Transform32/LConn1 -- Transform319/LConn1 -- Transform318/LConn1 -- Transform317/LConn1 -- Transform316/LConn1 -- Transform315/LConn1 -- Transform314/LConn1 -- Transform313/LConn1 -- Transform312/LConn1 -- ReferenceFrame/RConn1 -- F/RConn1 -- Transform311/LConn1 -- Transform310/LConn1 -- Transform31/LConn1 -- Transform309/LConn1 -- Transform308/LConn1 -- Transform307/LConn1 -- Transform306/LConn1 -- Transform305/LConn1 -- Transform304/LConn1 -- Transform303/LConn1 -- Transform302/LConn1 -- Transform301/LConn1 -- Transform300/LConn1 -- Transform30/LConn1 -- Transform3/LConn1 -- Transform299/LConn1 -- Transform298/LConn1 -- Transform297/LConn1 -- Transform296/LConn1 -- Transform295/LConn1 -- Transform294/LConn1 -- Transform293/LConn1 -- Transform292/LConn1 -- Transform291/LConn1 -- Transform290/LConn1 -- Transform29/LConn1 -- Transform289/LConn1 -- Transform288/LConn1 -- Transform287/LConn1 -- Transform286/LConn1 -- Transform285/LConn1 -- Transform284/LConn1 -- Transform283/LConn1 -- Transform282/LConn1 -- Transform281/LConn1 -- Transform280/LConn1 -- Transform28/LConn1 -- Transform279/LConn1 -- Transform278/LConn1 -- Transform277/LConn1 -- Transform276/LConn1 -- Transform275/LConn1 -- Transform274/LConn1 -- Transform273/LConn1 -- Transform272/LConn1 -- Transform271/LConn1 -- Transform270/LConn1 -- Transform27/LConn1 -- Transform269/LConn1 -- Transform268/LConn1 -- Transform267/LConn1 -- Transform266/LConn1 -- Transform265/LConn1 -- Transform264/LConn1 -- Transform263/LConn1 -- Transform262/LConn1 -- Transform261/LConn1 -- Transform260/LConn1 -- Transform26/LConn1 -- Transform259/LConn1 -- Transform258/LConn1 -- Transform257/LConn1 -- Transform256/LConn1 -- Transform255/LConn1 -- Transform254/LConn1 -- Transform253/LConn1 -- Transform252/LConn1 -- Transform251/LConn1 -- Transform250/LConn1 -- Transform25/LConn1 -- Transform249/LConn1 -- Transform248/LConn1 -- Transform247/LConn1 -- Transform246/LConn1 -- Transform245/LConn1 -- Transform244/LConn1 -- Transform243/LConn1 -- Transform242/LConn1 -- Transform241/LConn1 -- Transform240/LConn1 -- Transform24/LConn1 -- Transform239/LConn1 -- Transform238/LConn1 -- Transform237/LConn1 -- Transform236/LConn1 -- Transform235/LConn1 -- Transform234/LConn1 -- Transform233/LConn1 -- Transform232/LConn1 -- Transform231/LConn1 -- Transform230/LConn1 -- Transform23/LConn1 -- Transform229/LConn1 -- Transform228/LConn1 -- Transform227/LConn1 -- Transform226/LConn1 -- Transform225/LConn1 -- Transform224/LConn1 -- Transform223/LConn1 -- Transform222/LConn1 -- Transform221/LConn1 -- Transform220/LConn1 -- Transform22/LConn1 -- Transform219/LConn1 -- Transform218/LConn1 -- Transform217/LConn1 -- Transform216/LConn1 -- Transform215/LConn1 -- Transform214/LConn1 -- Transform213/LConn1 -- Transform212/LConn1 -- Transform211/LConn1 -- Transform210/LConn1 -- Transform21/LConn1 -- Transform209/LConn1 -- Transform208/LConn1 -- Transform207/LConn1 -- Transform206/LConn1 -- Transform205/LConn1 -- Transform204/LConn1 -- Transform203/LConn1 -- Transform202/LConn1 -- Transform201/LConn1 -- Transform200/LConn1 -- Transform20/LConn1 -- Transform2/LConn1 -- Transform199/LConn1 -- Transform198/LConn1 -- Transform197/LConn1 -- Transform196/LConn1 -- Transform195/LConn1 -- Transform194/LConn1 -- Transform193/LConn1 -- Transform192/LConn1 -- Transform191/LConn1 -- Transform190/LConn1 -- Transform19/LConn1 -- Transform189/LConn1 -- Transform188/LConn1 -- Transform187/LConn1 -- Transform186/LConn1 -- Transform185/LConn1 -- Transform184/LConn1 -- Transform183/LConn1 -- Transform182/LConn1 -- Transform181/LConn1 -- Transform180/LConn1 -- Transform18/LConn1 -- Transform179/LConn1 -- Transform178/LConn1 -- Transform177/LConn1 -- Transform176/LConn1 -- Transform175/LConn1 -- Transform174/LConn1 -- Transform173/LConn1 -- Transform172/LConn1 -- Transform171/LConn1 -- Transform170/LConn1 -- Transform17/LConn1 -- Transform169/LConn1 -- Transform168/LConn1 -- Transform167/LConn1 -- Transform166/LConn1 -- Transform165/LConn1 -- Transform164/LConn1 -- Transform163/LConn1 -- Transform162/LConn1 -- Transform161/LConn1 -- Transform160/LConn1 -- Transform16/LConn1 -- Transform159/LConn1 -- Transform158/LConn1 -- Transform157/LConn1 -- Transform156/LConn1 -- Transform155/LConn1 -- Transform154/LConn1 -- Transform153/LConn1 -- Transform152/LConn1 -- Transform151/LConn1 -- Transform150/LConn1 -- Transform15/LConn1 -- Transform149/LConn1 -- Transform148/LConn1 -- Transform147/LConn1 -- Transform146/LConn1 -- Transform145/LConn1 -- Transform144/LConn1 -- Transform143/LConn1 -- Transform142/LConn1 -- Transform141/LConn1 -- Transform140/LConn1 -- Transform14/LConn1 -- Transform139/LConn1 -- Transform138/LConn1 -- Transform137/LConn1 -- Transform136/LConn1 -- Transform135/LConn1 -- Transform134/LConn1 -- Transform133/LConn1 -- Transform132/LConn1 -- Transform131/LConn1 -- Transform130/LConn1 -- Transform13/LConn1 -- Transform129/LConn1 -- Transform128/LConn1 -- Transform127/LConn1 -- Transform126/LConn1 -- Transform125/LConn1 -- Transform124/LConn1 -- Transform123/LConn1 -- Transform122/LConn1 -- Transform121/LConn1 -- Transform120/LConn1 -- Transform12/LConn1 -- Transform119/LConn1 -- Transform118/LConn1 -- Transform117/LConn1 -- Transform116/LConn1 -- Transform115/LConn1 -- Transform114/LConn1 -- Transform113/LConn1 -- Transform112/LConn1 -- Transform111/LConn1 -- Transform110/LConn1 -- Transform11/LConn1 -- Transform109/LConn1 -- Transform108/LConn1 -- Transform107/LConn1 -- Transform106/LConn1 -- Transform105/LConn1 -- Transform104/LConn1 -- Transform103/LConn1 -- Transform102/LConn1 -- Transform101/LConn1 -- Transform100/LConn1 -- Transform10/LConn1 -- Transform1/LConn1
  Transform48/RConn1 -- mandUD_Hekimhan_Madencilik_ergnler_3028sasidik3_IGS_1_RIGID/LConn1
  M5_MirrorModel_004_05_1_IGS_1_RIGID/LConn1 -- Transform49/RConn1
  Transform5/RConn1 -- su_tanki_ayai_IGS_1_RIGID/LConn1
  MirrorPart4M5_Model_004_merkez_IGS_1_RIGID/LConn1 -- Transform50/RConn1
  Part5M5_Model_004_merkez_IGS_1_RIGID/LConn1 -- Transform51/RConn1
  Part3M5_Model_004_merkez_IGS_1_RIGID/LConn1 -- Transform52/RConn1
  MirrorPart5M5_Model_004_merkez_IGS_1_RIGID/LConn1 -- Transform53/RConn1
  M5_MirrorModel_004_Ayna_01_IGS_1_RIGID/LConn1 -- Transform54/RConn1
  MirrorPart3M5_Model_004_merkez_IGS_1_RIGID/LConn1 -- Transform55/RConn1
  M5_UV_01_IGS_1_RIGID/LConn1 -- Transform56/RConn1
  Transform57/RConn1 -- mandUD_Hekimhan_Madencilik_ergnler_3028arka_kapama_sac_IGS_1_RI/LConn1
  Transform58/RConn1 -- mandUD_Hekimhan_Madencilik_ergnler_3028ase_u_kapama_IGS_1_RIGID/LConn1
  Transform59/RConn1 -- mandUD_Hekimhan_Madencilik_ergnler_3028sasidik1_IGS_1_RIGID/LConn1
  Transform6/RConn1 -- x132zbmut4900zT13124_ozaas_Part1_IGS_4_RIGID/LConn1
  Transform60/RConn1 -- mandUD_Hekimhan_Madencilik_ergnler_3028sasidik2_IGS_1_RIGID/LConn1
  Transform61/RConn1 -- mandUD_Hekimhan_Madencilik_ergnler_3028sasidik4_IGS_1_RIGID/LConn1
  Transform62/RConn1 -- mandUD_Hekimhan_Madencilik_ergnler_3028asi_apraz_profil_IGS_1_R/LConn1
  Transform63/RConn1 -- mandUD_Hekimhan_Madencilik_ergnler_3028asi_u_kros_IGS_1_RIGID/LConn1
  Transform64/RConn1 -- mandUD_Hekimhan_Madencilik_ergnler_3028ase_U_kros_bayra_IGS_1_R/LConn1
  Transform65/RConn1 -- mandUD_Hekimhan_Madencilik_ergnler_3028asi_apraz_profil_2_IGS_1/LConn1
  Transform66/RConn1 -- mandUD_Hekimhan_Madencilik_ergnler_3028kulak_burcu_IGS_2_RIGID/LConn1
  Transform67/RConn1 -- mandUD_Hekimhan_Madencilik_ergnler_3028ase_U_kros_bayra_IGS_2_R/LConn1
  Transform68/RConn1 -- mandUD_Hekimhan_Madencilik_ergnler_3028ase_aprazlar_n_destek_IG/LConn1
  Transform69/RConn1 -- mandUD_Hekimhan_Madencilik_ergnler_3028papatya_IGS_2_RIGID/LConn1
  Transform7/RConn1 -- alminyumprofil2150_IGS_1_RIGID/LConn1
  Transform70/RConn1 -- mandUD_Hekimhan_Madencilik_ergnler_3028papatyann_kardei_IGS_1_R/LConn1
  Transform71/RConn1 -- mandUD_Hekimhan_Madencilik_ergnler_3028ase_n_destek_IGS_1_RIGID/LConn1
  Transform72/RConn1 -- mandUD_Hekimhan_Madencilik_ergnler_3028ase_U_kros_bayra_IGS_4_R/LConn1
  Transform73/RConn1 -- mandUD_Hekimhan_Madencilik_ergnler_3028ase_U_kros_bayra_IGS_3_R/LConn1
  Transform74/RConn1 -- mandUD_Hekimhan_Madencilik_ergnler_3028asi_apraz_profil_2_IGS_2/LConn1
  Transform75/RConn1 -- mandUD_Hekimhan_Madencilik_ergnler_3028ase_aprazlar_n_destek_2_/LConn1
  Transform76/RConn1 -- mandUD_Hekimhan_Madencilik_ergnler_3028kulak_burcu_IGS_1_RIGID/LConn1
  Transform77/RConn1 -- mandUD_Hekimhan_Madencilik_ergnler_3028papatya_IGS_1_RIGID/LConn1
  Transform78/RConn1 -- mandUD_Hekimhan_Madencilik_ergnler_3028ase_n_destek_IGS_2_RIGID/LConn1
  Transform79/RConn1 -- mandUD_Hekimhan_Madencilik_Mirrorergnler_3028U_ase_IGS_1_RIGID/LConn1
  Transform8/RConn1 -- x132zbmut4900zT13124_ozaas_Part1_IGS_3_RIGID/LConn1
  Transform80/RConn1 -- mandUD_Hekimhan_Madencilik_ergnler_3028papatyann_kardei_IGS_2_R/LConn1
  Transform81/RConn1 -- mandUD_Volvo_kutu_volvo_p1_IGS_1_RIGID/LConn1
  Transform82/RConn1 -- mandUD_Volvo_kutu_CH806_IGS_2_RIGID/LConn1
  Transform83/RConn1 -- mandUD_Hekimhan_Madencilik_ergnler_3028papatyann_kardei_IGS_3_R/LConn1
  Transform84/RConn1 -- mandUD_Volvo_kutu_CH806_IGS_1_RIGID/LConn1
  Transform85/RConn1 -- mandUD_Hekimhan_Madencilik_Mirrorergnler_3028ase_u_kapama_IGS_1/LConn1
  Transform86/RConn1 -- mandUD_Hekimhan_Madencilik_1yg01_IGS_1_RIGID/LConn1
  Transform87/RConn1 -- mandUD_Volvo_kutu_CH805_IGS_1_RIGID/LConn1
  Transform88/RConn1 -- mandUD_Volvo_kutu_CH805_IGS_2_RIGID/LConn1
  Transform89/RConn1 -- mandUD_Volvo_kutu_volvo_p3_IGS_1_RIGID/LConn1
  Transform9/RConn1 -- alminyumprofil2150_IGS_3_RIGID/LConn1
  Transform90/RConn1 -- mandUD_Volvo_kutu_volvo_p5_IGS_1_RIGID/LConn1
  Transform91/RConn1 -- mandUD_Hekimhan_Madencilik_ergnler_3028papatyann_kardei_IGS_4_R/LConn1
  M5_erp33360_kilit_paras_aya_IGS_1_RIGID/LConn1 -- Transform92/RConn1
  M5_erp33360_kilit_paras_aya_IGS_2_RIGID/LConn1 -- Transform93/RConn1
  M5_erp33360_kilit_burc_2_IGS_2_RIGID/LConn1 -- Transform94/RConn1
  M5_erp33360_kilit_mil_IGS_1_RIGID/LConn1 -- Transform95/RConn1
  M5_erp33360_mekanik_kapak_kilit_paras_IGS_1_RIGID/LConn1 -- Transform96/RConn1
  M5_erp33360_BUR2_IGS_1_RIGID/LConn1 -- Transform97/RConn1
  M5_erp33360_Kapak_alt_kapama_IGS_1_RIGID/LConn1 -- Transform98/RConn1
  M5_erp33360_sallama_ayak_IGS_1_RIGID/LConn1 -- Transform99/RConn1
